simulink model "motor"  (R2024b)
settings: Solver=VariableStepAuto  StartTime=0.0  StopTime=10  RelTol=1e-3
undefined symbols (not defined in the file or in its folder): kt, kv, Vnom
libraries: cstblocks x2
settings Model: Creator=turco  LastModifiedBy=turco

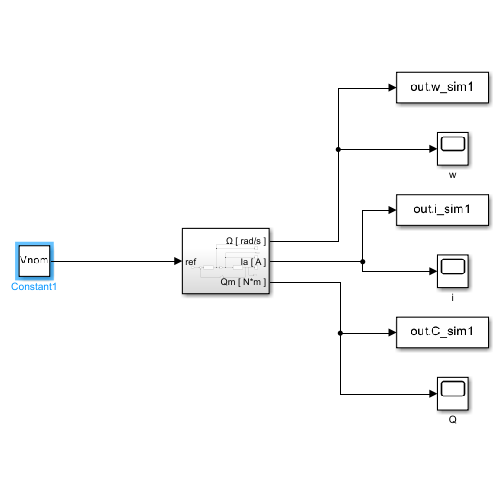
[thumbnail: Simulink's stored preview of the top-level diagram]
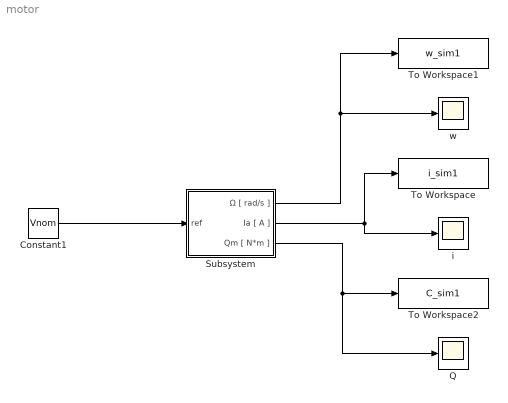
== system motor ==
  Constant1 : Constant  Value=Vnom
  Q : Scope
  Subsystem : Subsystem
  To Workspace : ToWorkspace  VariableName=i_sim1  SaveFormat=Timeseries  SampleTime=-1
  To Workspace1 : ToWorkspace  VariableName=w_sim1  SaveFormat=Timeseries  SampleTime=-1
  To Workspace2 : ToWorkspace  VariableName=C_sim1  SaveFormat=Timeseries  SampleTime=-1
  i : Scope
  w : Scope
  wires:
  Subsystem/1(Ω [ rad/s ]) -> To Workspace1/1, w/1
  Subsystem/2(Ia [ A ]) -> i/1, To Workspace/1
  Subsystem/3(Qm [ N*m ]) -> Q/1, To Workspace2/1
  Constant1/1 -> Subsystem/1(ref)

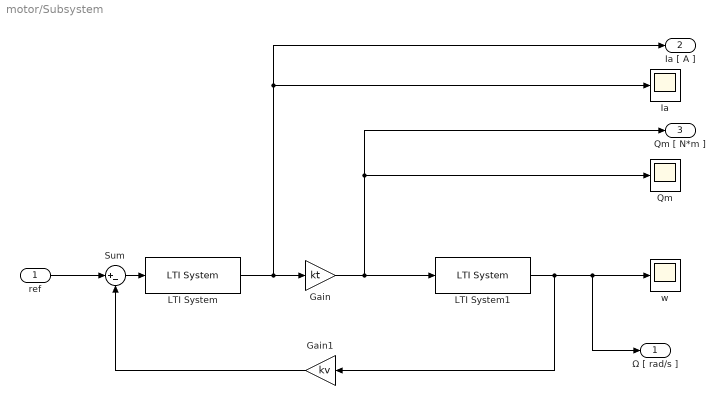
== system motor/Subsystem ==
  ref : Inport
  Gain : Gain  Gain=kt
  Gain1 : Gain  Gain=kv
  Ia : Scope
  LTI System : cstblocks/LTI System  sys=Pel  IC=[]  PadeOrder=0
  LTI System1 : cstblocks/LTI System  sys=Pmec  IC=[]  PadeOrder=0
  "Qm " : Scope
  Sum : Sum  Inputs=|+-
  w : Scope
  Ω [ rad/s ] : Outport
  Ia [ A ] : Outport  Port=2
  Qm [ N*m ] : Outport  Port=3
  wires:
  LTI System1/1 -> Ω [ rad/s ]/1, w/1, Gain1/1
  Gain1/1 -> Sum/2
  Gain/1 -> Qm [ N*m ]/1, "Qm "/1, LTI System1/1
  Sum/1 -> LTI System/1
  LTI System/1 -> Ia [ A ]/1, Ia/1, Gain/1
  ref/1 -> Sum/1
